simulink library "Stewart_Gough_Library"  (Simulink 7.7)
settings: Solver=ode45  StartTime=0.0  StopTime=10.0  RelTol=1e-3
undefined symbols (not defined in the file or in its folder): Aa1, Bb1, Cc1, Com1, Dd1, Dis_motor, none
libraries: simulink x13, Diamond16AT_UNAL x3, xpcseriallib x2, Stewart_Gough_Library x1
settings Model: Creator=BolivarNieto  LastModifiedBy=Edgar

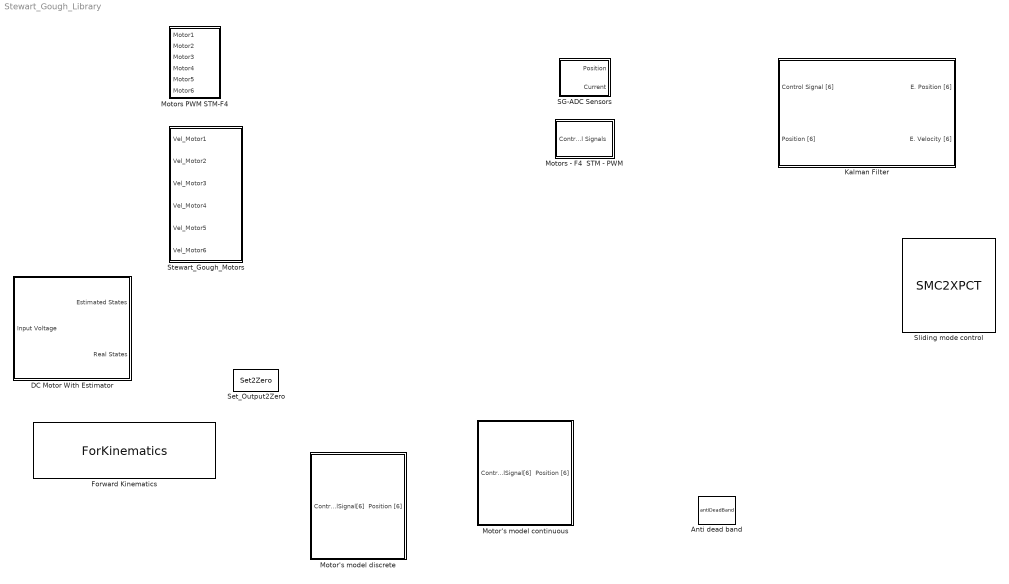
== system Stewart_Gough_Library ==
  Anti dead band : S-Function  FunctionName=antiDeadBand  Parameters=SampleTime,AntiDeadBand  EnableBusSupport=off  mask{AntiDeadBand=20, SampleTime=-1}
      mask prompts: AntiDeadBand "Anti dead band offset"; SampleTime "Sample Time (-1 inherit sample time)"
      mask Display:
      | plot([0 10],[0 10])
      | plot([10 10],[10 30])
      | plot([10 20],[30 40])
  DC Motor With Estimator : Subsystem  mask(DC Motor dynamic model){tau_m=0, kdc_m=0, iniVelo_m=0, iniPos_m=0, V_m=0}
      mask prompts: tau_m "Motor Tau"; kdc_m "Motor Kdc"; iniVelo_m "Initial Velocity"; iniPos_m "Initial Position"; V_m "Estimation Vector"
      mask help: DC Motor dynamic model with saturation, dead band, saturation, Band-Limited white noise and full state estimator
  Forward Kinematics : S-Function  FunctionName=ForKinematics  Parameters=SGini.ai,SGini.bi,ActOff  EnableBusSupport=off  mask(Forward Kinematics - Stewart Gough platform){AngBase=20, AngMobi=30, RadBase=0.150, RadMobi=0.090, ActMax=0.74676, ActMin=0.44196, ActOff=0.5486, OffZBase=0.066, OffZMobile=0.0409082}
      mask prompts: AngBase "Angle between group of joints - Base (Deg)"; AngMobi "Angle between group of joints - Mobile (Deg)"; RadBase "Radious base (m)"; RadMobi "Radious mobile (m)"; ActMax "Actuator max (m)"; ActMin "Actuator min (m)"; ActOff "Actuator Offset (m)"; OffZBase "Offset Z - Base (m)"; OffZMobile "Offset Z - Mobile (m)"
      mask init:
      | AngBase = AngBase/2;
      | 
      | tmpAnglBase = [AngBase;120-AngBase;120+AngBase;240-AngBase;240+AngBase;360-AngBase]*pi/180; %Angular arrangement of joints
      | 
      | aA = zeros(3,6);
      | for i=1:6
      |     aA(:,i)=[sin(tmpAnglBase(i))*RadBase;cos(tmpAnglBase(i))*RadBase; OffZBase];
      | end
      | 
      | AngMobi = AngMobi/2;
      | 
      | tmpAnglMobi = [60-AngMobi;60+AngMobi;180-AngMobi;180+AngMobi;300-AngMobi;300+AngMobi]*pi/180; %Angular arrangement of joints
      | 
      | bB = zeros(3,6);
      | for i=1:6
      |     bB(:,i)=[sin(tmpAnglMobi(i))*RadMobi;cos(tmpAnglMobi(i))*RadMobi; -OffZMobile];
      | end
      | 
      | SGini.ai = aA;
      | SGini.bi = bB;
      mask TabNameString: SG Parameters,SG Parameters,SG Parameters,SG Parameters,SG Parameters,SG Parameters,SG Parameters,SG Parameters,SG Parameters
      mask Display:
      | port_label('output', 1, 'Position WS [6]')
      | fprintf('OUTPUT \n UNITS: \n XYZ (mts) \n RPY (rad)')
      | port_label('input', 1, 'Position [6] (mts)')
  Kalman Filter : Subsystem  mask(Kalman filter){Qin=[2,2,2,2,2,2], Rin=[1,1,1,1,1,1]*1e-6, IniPos=[70,70,70,70,70,70], IniVel=[0,0,0,0,0,0], SamTimeKal=0.001}
      mask prompts: Qin "Covariance vector of white process noise w, Q [1x6]:"; Rin "Covariance vector of white measurement noise v, R [1x6]:"; IniPos "Vector of initial position (mm) [1x6]:"; IniVel "Vector of initial velocity (mm/s) [1x6]:"; SamTimeKal "Sample Time:"
      mask help:
      | Firgelli actuator's Kalman filter.
      |     --Q: [1x6] vector with the white process noise covariance, it is relative to R and measures the quality of the model compared to the sensor.
      |     --R: [1x6] vector with the white measurement noise covariance, it is relative to Q and measures the quality of the sensor compared to the model.
      mask init:
      | %-------------------------------Actuators' parameters
      | tau(1)=12.9;    %min
      | tau(2)=20.9;
      | tau(3)=16;
      | tau(4)=26.2;    %max
      | tau(5)=17.1;
      | tau(6)=15.2;    
      | 
      | kdc(1)=35.737;  %min
      | kdc(2)=65.089;
      | kdc(3)=51.966;
      | kdc(4)=74.788;  %max
      | kdc(5)=49.788;
      | kdc(6)=51.427;
      | 
      | %--------------------------------NUMBER OF ACTUATOR
      | i=1;
      | tauT=tau(i);
      | kdcT=kdc(i);
      | %--------------------------------Steady state representation
      | A=[0 1;0 -tauT];
      | B=[0;kdcT];
      | C=[1 0];
      | D=0;
      | G=[0;1];             %Process noise (noise at the input of the )
      | H=0;
      | 
      | Aa=A;
      | Bb=[B G];
      | Cc=C;
      | Dd=[D H];
      | 
      | Motor = ss(Aa,Bb,Cc,Dd);             %DC-Motor second order
      | %--------------------------------Kalman design
      | N=0;
      | [kest,L,P] = kalman(Motor,Qin(i),Rin(i),N);
      | KalmanDis1=c2d(kest,SamTimeKal);
      | 
      | %--------------------------------NUMBER OF ACTUATOR
      | i=2;
      | tauT=tau(i);
      | kdcT=kdc(i);
      | %--------------------------------Steady state representation
      | A=[0 1;0 -tauT];
      | B=[0;kdcT];
      | C=[1 0];
      | D=0;
      | G=[0;1];             %Process noise (noise at the input of the )
      | H=0;
      | 
      | Aa=A;
      | Bb=[B G];
      | Cc=C;
      | Dd=[D H];
      | 
      | Motor = ss(Aa,Bb,Cc,Dd);             %DC-Motor second order
      | %--------------------------------Kalman design
      | N=0;
      | [kest,L,P] = kalman(Motor,Qin(i),Rin(i),N);
      | KalmanDis2=c2d(kest,SamTimeKal);
      | 
      | %--------------------------------NUMBER OF ACTUATOR
      | i=3;
      | tauT=tau(i);
      | kdcT=kdc(i);
      | %--------------------------------Steady state representation
      | A=[0 1;0 -tauT];
      | B=[0;kdcT];
      | C=[1 0];
      | D=0;
      | G=[0;1];             %Process noise (noise at the input of the )
      | H=0;
      | 
      | Aa=A;
      | Bb=[B G];
      | Cc=C;
      | Dd=[D H];
      | 
      | Motor = ss(Aa,Bb,Cc,Dd);             %DC-Motor second order
      | %--------------------------------Kalman design
      | N=0;
      | [kest,L,P] = kalman(Motor,Qin(i),Rin(i),N);
      | KalmanDis3=c2d(kest,SamTimeKal);
      | 
      | %--------------------------------NUMBER OF ACTUATOR
      | i=4;
      | tauT=tau(i);
      | kdcT=kdc(i);
      | %--------------------------------Steady state representation
      | A=[0 1;0 -tauT];
      | B=[0;kdcT];
      | C=[1 0];
      | D=0;
      | G=[0;1];             %Process noise (noise at the input of the )
      | H=0;
      | 
      | Aa=A;
      | Bb=[B G];
      | Cc=C;
      | Dd=[D H];
      | 
      | Motor = ss(Aa,Bb,Cc,Dd);             %DC-Motor second order
      | %--------------------------------Kalman design
      | N=0;
      | [kest,L,P] = kalman(Motor,Qin(i),Rin(i),N);
      | KalmanDis4=c2d(kest,SamTimeKal);
      | 
      | %--------------------------------NUMBER OF ACTUATOR
      | i=5;
      | tauT=tau(i);
      | kdcT=kdc(i);
      | %--------------------------------Steady state representation
      | A=[0 1;0 -tauT];
      | B=[0;kdcT];
      | C=[1 0];
      | D=0;
      | G=[0;1];             %Process noise (noise at the input of the )
      | H=0;
      | 
      | Aa=A;
      | Bb=[B G];
      | Cc=C;
      | Dd=[D H];
      | 
      | Motor = ss(Aa,Bb,Cc,Dd);             %DC-Motor second order
      | %--------------------------------Kalman design
      | N=0;
      | [kest,L,P] = kalman(Motor,Qin(i),Rin(i),N);
      | KalmanDis5=c2d(kest,SamTimeKal);
      | 
      | %--------------------------------NUMBER OF ACTUATOR
      | i=6;
      | tauT=tau(i);
      | kdcT=kdc(i);
      | %--------------------------------Steady state representation
      | A=[0 1;0 -tauT];
      | B=[0;kdcT];
      | C=[1 0];
      | D=0;
      | G=[0;1];             %Process noise (noise at the input of the )
      | H=0;
      | 
      | Aa=A;
      | Bb=[B G];
      | Cc=C;
      | Dd=[D H];
      | 
      | Motor = ss(Aa,Bb,Cc,Dd);             %DC-Motor second order
      | %--------------------------------Kalman design
      | N=0;
      | [kest,L,P] = kalman(Motor,Qin(i),Rin(i),N);
      | KalmanDis6=c2d(kest,SamTimeKal);
      mask Display:
      | disp('Estimator \n Firgelli Actuator')
      | port_label('output', 1, 'E. Position [6]')
      | port_label('output', 2, 'E. Velocity [6]')
      | port_label('input', 1, 'Control Signal [6]')
      | port_label('input', 2, 'Position [6]')
  Motor's model continuous : Subsystem  mask{Taus=[12.9;20.9;16;26.2;17.1;15.2], Kdcs=[35.737; 65.089; 51.966; 74.788; 49.788; 51.427], IniPos=[70;70;70;70;70;70], IniVel=[0;0;0;0;0;0], Vmax=12}
      mask prompts: Taus "Tau:"; Kdcs "Kdc:"; IniPos "Initial Position vector:"; IniVel "Initial Velocity vector:"; Vmax "Motor peak Voltage:"
  Motor's model discrete : Subsystem  mask{Taus=[12.9;20.9;16;26.2;17.1;15.2], Kdcs=[35.737; 65.089; 51.966; 74.788; 49.788; 51.427], IniPos=[70;70;70;70;70;70], IniVel=[0;0;0;0;0;0], Vmax=12}
      mask prompts: Taus "Tau:"; Kdcs "Kdc:"; IniPos "Initial position vector:"; IniVel "Initial Velocity Vector"; Vmax "Motor peak Voltage"
      mask init:
      | for i = 1:6
      |     A = [0 1; 0 -Taus(i)];
      |     B = [0; Kdcs(i)];
      |     C = [1 0;0 1];
      |     D = [0;0];    
      |     Con_motor(:,:,i) = ss(A,B,C,D);
      |     Dis_motor(:,:,i) = c2d(Con_motor(:,:,i),0.001);
      | end
  Motors - F4  STM - PWM : Subsystem  RequirementInfo="{}  %GIDa_83dcfb88_5bb3_4bf6_bc9f_f3909d4bf5a3"
      mask Type: Protocol for PWM generation through STM-F4
      mask Description:
      | Comunication protocol for PWM generation. This block communicates a STM-F4 through serial comunication. The STM-F4 generates the PWMs required for motor control.
      | 
      | The input for this block is the percentage duty cicle for each of the six motors.
  Motors PWM STM-F4 : Subsystem  mask(Protocol for PWM generation through a STM-F4 board){Satura=80}
      mask prompts: Satura "Saturation"
      mask help:
      | Comunication protocol for PWM generation. This block communicates a STM-F4 through serial comunication. The STM-F4 generates the PWMs required for motor control.
      |
      | The input for this block is the percentage duty cicle for each of the six motors.
      mask Help: No Help!! ahhhh!!
  SG-ADC Sensors : Subsystem  mask(SG-ADC-Sensors){SamTimeADC=0.001, CutFreq=20, IniSt=[0 0 0 0 0 0]}
      mask prompts: SamTimeADC "Sample Time"; CutFreq "Cutoff frequency"; IniSt "Initial States Filter:"
      mask help: ADC from sensors, reading from I/O board daemmond 16AT and using a Discrete digital filter to remove noise.
      mask init:
      | IniStates=[0 IniSt(1)*1.4141;...
      |            0 IniSt(2)*1.4141;...
      |            0 IniSt(3)*1.4141;...
      |            0 IniSt(4)*1.4141;...
      |            0 IniSt(5)*1.4141;...
      |            0 IniSt(6)*1.4141;...                
      |            ];
      | %Filter design
      | n=2;
      | freq=1/SamTimeADC;
      | Wn=CutFreq/(freq/2);          %Sampled to 1kHz and cutof frequency of 20Hz
      | [Aa1,Bb1,Cc1,Dd1]=butter(n,Wn,'low');
      mask TabNameString: Main,Main,Main
  Set_Output2Zero : S-Function  FunctionName=Set2Zero  EnableBusSupport=off
  Sliding mode control : S-Function  FunctionName=SMC2XPCT  Parameters=eta, lambda, tau  EnableBusSupport=off  mask(Sliding mode control block){eta=0.1, lambda=1, tau=26.2}
      mask help:
      | This block implements a Sliding Mode position controler for a DC-motor.
      | It requieres the motor's position and velocity along with the desired position, velocity and aceleration.
      |
      | --Eta: Is related to a "safe factor" for stability.
      | --Lambda: Determines the rate of convergence to 0 of the error.
      | --Tau: Refers to the coeficient tau in the dinamic model.
      |
      | To change especific constants like F, please go to the "mdlOutputs" function in the c code of the S-function.
      mask Display:
      | port_label('output', 1, 'U')
      | port_label('output', 2, 'S')
      | port_label('input', 1, 'xd, xdP, xdPP')
      | port_label('input', 2, 'dm, dmP')
      | disp('SMC')
  Stewart_Gough_Motors : Subsystem  mask(Stewart Gough Motors Block  ){PWM_amp=4, PWM_freq=1000, Rpm2Pwm=1, SampleTime_ed=0.00005}
      mask prompts: PWM_amp "PWM Amplitude"; PWM_freq "PWM frequency (Hz)"; Rpm2Pwm "RPM to PWM's duty cycle gain"; SampleTime_ed "SampleTime"
      mask help: PWM Generator for 6 motors at the Stewart Gough. PWM generation is compatible with the H-Bridge 33887
      mask Help:
      | Set PWM parameters from the block dialog:
      | 
      | * PWM Amplitude stands for the amplitude when PWM is at high.
      | * RPM to PWM's duty cycle sets the conversion gain between the motor speed in RPM and the correspond duty cycle at the PWM generation.

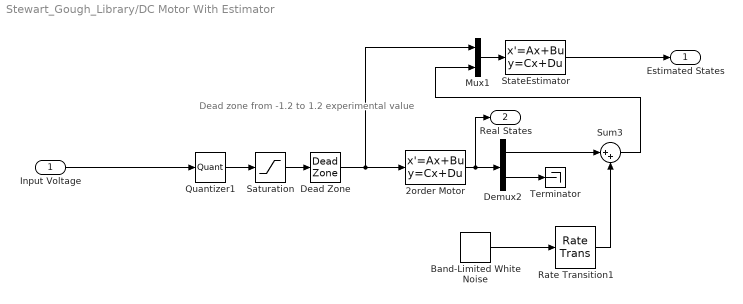
== system Stewart_Gough_Library/DC Motor With Estimator ==
  note: Dead zone from -1.2 to 1.2
      | experimental value
  Input Voltage : Inport
  2order Motor : StateSpace  A=[0 1; 0 -tau_m]  B=[0; kdc_m]  C=[1 0;0 1]  D=[0;0]  X0=[iniPos_m iniVelo_m]  ContinuousStateAttributes={'LinearPosition','LinearVelocity'}
  Band-Limited White Noise : simulink/Sources/Band-Limited White Noise  SystemSampleTime=-1  Cov=[0.0001]  Ts=0.1  seed=[23341]
  Dead Zone : DeadZone  LowerValue=0  UpperValue=0  ZeroCross=off  SaturateOnIntegerOverflow=on
  Demux2 : Demux  Outputs=2
  Mux1 : Mux  Inputs=2
  Quantizer1 : Quantizer  QuantizationInterval=0.1
  Rate Transition1 : RateTransition
  Saturation : Saturate  UpperLimit=12  LowerLimit=-12  ZeroCross=off
  StateEstimator : StateSpace  A=[-V_m(1) 1; -V_m(2) -tau_m]  B=[0 V_m(1); kdc_m V_m(2)]  C=[1 0; 0 1]  D=[0 0; 0 0]  X0=[iniPos_m iniVelo_m]  ContinuousStateAttributes={'LinearPositionEstimated','LinearVelocityEstimated'}
  Sum3 : Sum  Inputs=|++
  Terminator : Terminator
  Estimated States : Outport
  Real States : Outport  Port=2
  wires:
  Sum3/1 -> Mux1/2
  Mux1/1 -> StateEstimator/1
  Input Voltage/1 -> Quantizer1/1
  Dead Zone/1 -> 2order Motor/1, Mux1/1
  Saturation/1 -> Dead Zone/1
  Quantizer1/1 -> Saturation/1
  Rate Transition1/1 -> Sum3/2
  Band-Limited White Noise/1 -> Rate Transition1/1
  2order Motor/1 -> Demux2/1, Real States/1
  Demux2/1 -> Sum3/1
  Demux2/2 -> Terminator/1
  StateEstimator/1 -> Estimated States/1

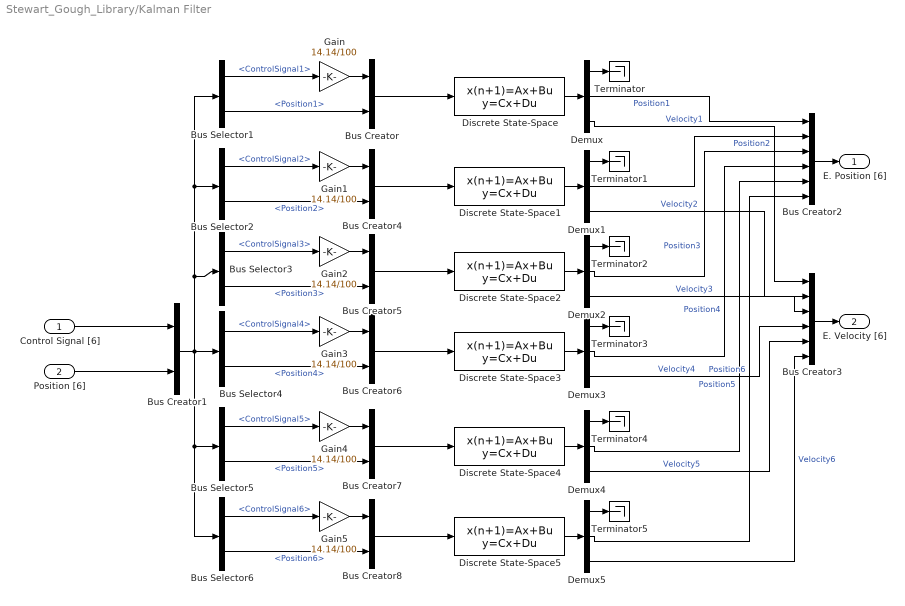
== system Stewart_Gough_Library/Kalman Filter ==
  Control Signal [6] : Inport
  Position [6] : Inport  Port=2
  Bus Creator{,1,4..8} (7 alike) : BusCreator  Inputs=2
  Bus Creator2 : BusCreator  Inputs=6
  Bus Creator3 : BusCreator  Inputs=6
  Bus Selector1 : BusSelector  OutputSignals=signal1.ControlSignal1,signal2.Position1
  Bus Selector2 : BusSelector  OutputSignals=signal1.ControlSignal2,signal2.Position2
  Bus Selector3 : BusSelector  OutputSignals=signal1.ControlSignal3,signal2.Position3
  Bus Selector4 : BusSelector  OutputSignals=signal1.ControlSignal4,signal2.Position4
  Bus Selector5 : BusSelector  OutputSignals=signal1.ControlSignal5,signal2.Position5
  Bus Selector6 : BusSelector  OutputSignals=signal1.ControlSignal6,signal2.Position6
  Demux{,1..5} (6 alike) : Demux  Outputs=3
  Discrete State-Space : DiscreteStateSpace  A=KalmanDis1.A  B=KalmanDis1.B  C=KalmanDis1.C  D=KalmanDis1.D  X0=[IniPos(1) IniVel(1)]  SampleTime=SamTimeKal
  Discrete State-Space1 : DiscreteStateSpace  A=KalmanDis2.A  B=KalmanDis2.B  C=KalmanDis2.C  D=KalmanDis2.D  X0=[IniPos(2) IniVel(2)]  SampleTime=SamTimeKal
  Discrete State-Space2 : DiscreteStateSpace  A=KalmanDis3.A  B=KalmanDis3.B  C=KalmanDis3.C  D=KalmanDis3.D  X0=[IniPos(3) IniVel(3)]  SampleTime=SamTimeKal
  Discrete State-Space3 : DiscreteStateSpace  A=KalmanDis4.A  B=KalmanDis4.B  C=KalmanDis4.C  D=KalmanDis4.D  X0=[IniPos(4) IniVel(4)]  SampleTime=SamTimeKal
  Discrete State-Space4 : DiscreteStateSpace  A=KalmanDis5.A  B=KalmanDis5.B  C=KalmanDis5.C  D=KalmanDis5.D  X0=[IniPos(5) IniVel(5)]  SampleTime=SamTimeKal
  Discrete State-Space5 : DiscreteStateSpace  A=KalmanDis6.A  B=KalmanDis6.B  C=KalmanDis6.C  D=KalmanDis6.D  X0=[IniPos(6) IniVel(6)]  SampleTime=SamTimeKal
  Gain{,1..5} (6 alike) : Gain  Gain=14.14/100
  Terminator{,1..5} (6 alike) : Terminator
  E. Position [6] : Outport
  E. Velocity [6] : Outport  Port=2
  wires:
  Bus Creator1/1 -> Bus Selector1/1, Bus Selector2/1, Bus Selector3/1, Bus Selector4/1, Bus Selector6/1, Bus Selector5/1
  Control Signal [6]/1 -> Bus Creator1/1
  Bus Creator2/1 -> E. Position [6]/1
  Position [6]/1 -> Bus Creator1/2
  Discrete State-Space/1 -> Demux/1
  Discrete State-Space1/1 -> Demux1/1
  Discrete State-Space2/1 -> Demux2/1
  Discrete State-Space3/1 -> Demux3/1
  Discrete State-Space4/1 -> Demux4/1
  Discrete State-Space5/1 -> Demux5/1
  Demux/1 -> Terminator/1
  Demux1/1 -> Terminator1/1
  Demux2/1 -> Terminator2/1
  Demux3/1 -> Terminator3/1
  Demux4/1 -> Terminator4/1
  Demux5/1 -> Terminator5/1
  Demux/2 -> Bus Creator2/1  "Position1"
  Demux1/2 -> Bus Creator2/2  "Position2"
  Demux2/2 -> Bus Creator2/3  "Position3"
  Demux3/2 -> Bus Creator2/4  "Position4"
  Demux4/2 -> Bus Creator2/5  "Position5"
  Demux5/2 -> Bus Creator2/6  "Position6"
  Bus Creator3/1 -> E. Velocity [6]/1
  Demux/3 -> Bus Creator3/1  "Velocity1"
  Demux1/3 -> Bus Creator3/2  "Velocity2"
  Demux2/3 -> Bus Creator3/3  "Velocity3"
  Demux3/3 -> Bus Creator3/4  "Velocity4"
  Demux5/3 -> Bus Creator3/6  "Velocity6"
  Demux4/3 -> Bus Creator3/5  "Velocity5"
  Bus Selector1/1 -> Gain/1  "<ControlSignal1>"
  Gain/1 -> Bus Creator/1
  Bus Selector1/2 -> Bus Creator/2  "<Position1>"
  Bus Creator/1 -> Discrete State-Space/1
  Gain1/1 -> Bus Creator4/1
  Bus Creator4/1 -> Discrete State-Space1/1
  Gain2/1 -> Bus Creator5/1
  Bus Creator5/1 -> Discrete State-Space2/1
  Gain3/1 -> Bus Creator6/1
  Gain4/1 -> Bus Creator7/1
  Gain5/1 -> Bus Creator8/1
  Bus Creator6/1 -> Discrete State-Space3/1
  Bus Creator7/1 -> Discrete State-Space4/1
  Bus Creator8/1 -> Discrete State-Space5/1
  Bus Selector2/1 -> Gain1/1  "<ControlSignal2>"
  Bus Selector2/2 -> Bus Creator4/2  "<Position2>"
  Bus Selector3/1 -> Gain2/1  "<ControlSignal3>"
  Bus Selector3/2 -> Bus Creator5/2  "<Position3>"
  Bus Selector4/1 -> Gain3/1  "<ControlSignal4>"
  Bus Selector4/2 -> Bus Creator6/2  "<Position4>"
  Bus Selector5/1 -> Gain4/1  "<ControlSignal5>"
  Bus Selector5/2 -> Bus Creator7/2  "<Position5>"
  Bus Selector6/1 -> Gain5/1  "<ControlSignal6>"
  Bus Selector6/2 -> Bus Creator8/2  "<Position6>"

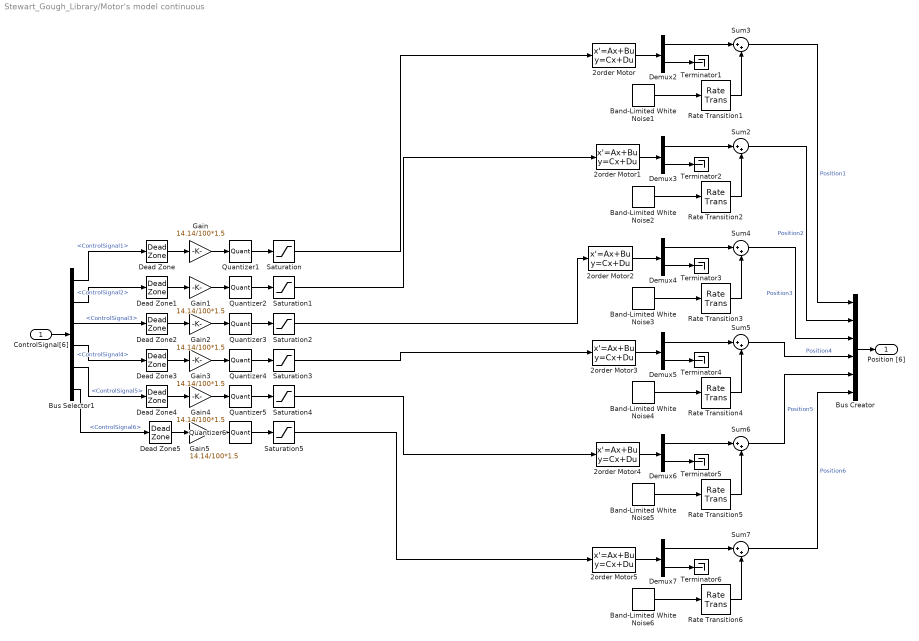
== system Stewart_Gough_Library/Motor's model continuous ==
  ControlSignal[6] : Inport
  2order Motor : StateSpace  A=[0 1; 0 -Taus(1)]  B=[0; Kdcs(1)]  C=[1 0;0 1]  D=[0;0]  X0=[IniPos(1) IniVel(1)]  ContinuousStateAttributes={'LinearPosition','LinearVelocity'}
  2order Motor1 : StateSpace  A=[0 1; 0 -Taus(2)]  B=[0; Kdcs(2)]  C=[1 0;0 1]  D=[0;0]  X0=[IniPos(2) IniVel(2)]  ContinuousStateAttributes={'LinearPosition','LinearVelocity'}
  2order Motor2 : StateSpace  A=[0 1; 0 -Taus(3)]  B=[0; Kdcs(3)]  C=[1 0;0 1]  D=[0;0]  X0=[IniPos(3) IniVel(3)]  ContinuousStateAttributes={'LinearPosition','LinearVelocity'}
  2order Motor3 : StateSpace  A=[0 1; 0 -Taus(4)]  B=[0; Kdcs(4)]  C=[1 0;0 1]  D=[0;0]  X0=[IniPos(4) IniVel(4)]  ContinuousStateAttributes={'LinearPosition','LinearVelocity'}
  2order Motor4 : StateSpace  A=[0 1; 0 -Taus(5)]  B=[0; Kdcs(5)]  C=[1 0;0 1]  D=[0;0]  X0=[IniPos(5) IniVel(5)]  ContinuousStateAttributes={'LinearPosition','LinearVelocity'}
  2order Motor5 : StateSpace  A=[0 1; 0 -Taus(6)]  B=[0; Kdcs(6)]  C=[1 0;0 1]  D=[0;0]  X0=[IniPos(6) IniVel(6)]  ContinuousStateAttributes={'LinearPosition','LinearVelocity'}
  Band-Limited White Noise{1..6} (6 alike) : simulink/Sources/Band-Limited White Noise  SystemSampleTime=-1  Cov=[0.0001]  Ts=0.1  seed=[23341]
  Bus Creator : BusCreator  Inputs=6
  Bus Selector1 : BusSelector  OutputSignals=ControlSignal1,ControlSignal2,ControlSignal3,ControlSignal4,ControlSignal5,ControlSignal6
  Dead Zone{,1..5} (6 alike) : DeadZone  LowerValue=-9.5  UpperValue=6  ZeroCross=off  SaturateOnIntegerOverflow=on
  Demux{2..7} (6 alike) : Demux  Outputs=2
  Gain{,1..5} (6 alike) : Gain  Gain=14.14/100*1.5
  Quantizer{1..6} (6 alike) : Quantizer  QuantizationInterval=0.1
  Rate Transition{1..6} (6 alike) : RateTransition
  Saturation{,1..5} (6 alike) : Saturate  UpperLimit=Vmax*1.25  LowerLimit=-Vmax*1.2  ZeroCross=off
  Sum{2..7} (6 alike) : Sum  Inputs=|++
  Terminator{1..6} (6 alike) : Terminator
  Position [6] : Outport
  wires:
  Demux2/2 -> Terminator1/1
  Demux2/1 -> Sum3/1
  2order Motor/1 -> Demux2/1
  Band-Limited White Noise1/1 -> Rate Transition1/1
  Rate Transition1/1 -> Sum3/2
  Saturation/1 -> 2order Motor/1
  Saturation2/1 -> 2order Motor2/1
  Saturation3/1 -> 2order Motor3/1
  Saturation4/1 -> 2order Motor4/1
  Saturation5/1 -> 2order Motor5/1
  Demux3/2 -> Terminator2/1
  Demux3/1 -> Sum2/1
  2order Motor1/1 -> Demux3/1
  Band-Limited White Noise2/1 -> Rate Transition2/1
  Rate Transition2/1 -> Sum2/2
  Demux4/2 -> Terminator3/1
  Demux4/1 -> Sum4/1
  2order Motor2/1 -> Demux4/1
  Band-Limited White Noise3/1 -> Rate Transition3/1
  Rate Transition3/1 -> Sum4/2
  Demux5/2 -> Terminator4/1
  Demux5/1 -> Sum5/1
  2order Motor3/1 -> Demux5/1
  Band-Limited White Noise4/1 -> Rate Transition4/1
  Rate Transition4/1 -> Sum5/2
  Demux6/2 -> Terminator5/1
  Demux6/1 -> Sum6/1
  2order Motor4/1 -> Demux6/1
  Band-Limited White Noise5/1 -> Rate Transition5/1
  Rate Transition5/1 -> Sum6/2
  Demux7/2 -> Terminator6/1
  Demux7/1 -> Sum7/1
  2order Motor5/1 -> Demux7/1
  Band-Limited White Noise6/1 -> Rate Transition6/1
  Rate Transition6/1 -> Sum7/2
  Sum3/1 -> Bus Creator/1  "Position1"
  Sum2/1 -> Bus Creator/2  "Position2"
  Sum4/1 -> Bus Creator/3  "Position3"
  Sum5/1 -> Bus Creator/4  "Position4"
  Sum6/1 -> Bus Creator/5  "Position5"
  Sum7/1 -> Bus Creator/6  "Position6"
  Bus Selector1/1 -> Dead Zone/1  "<ControlSignal1>"
  Bus Selector1/2 -> Dead Zone1/1  "<ControlSignal2>"
  Bus Selector1/3 -> Dead Zone2/1  "<ControlSignal3>"
  Bus Selector1/4 -> Dead Zone3/1  "<ControlSignal4>"
  Bus Selector1/5 -> Dead Zone4/1  "<ControlSignal5>"
  Bus Selector1/6 -> Dead Zone5/1  "<ControlSignal6>"
  ControlSignal[6]/1 -> Bus Selector1/1
  Bus Creator/1 -> Position [6]/1
  Saturation1/1 -> 2order Motor1/1
  Quantizer1/1 -> Saturation/1
  Quantizer2/1 -> Saturation1/1
  Quantizer3/1 -> Saturation2/1
  Quantizer4/1 -> Saturation3/1
  Quantizer5/1 -> Saturation4/1
  Quantizer6/1 -> Saturation5/1
  Gain/1 -> Quantizer1/1
  Gain1/1 -> Quantizer2/1
  Gain2/1 -> Quantizer3/1
  Gain3/1 -> Quantizer4/1
  Gain4/1 -> Quantizer5/1
  Gain5/1 -> Quantizer6/1
  Dead Zone1/1 -> Gain1/1
  Dead Zone2/1 -> Gain2/1
  Dead Zone3/1 -> Gain3/1
  Dead Zone4/1 -> Gain4/1
  Dead Zone5/1 -> Gain5/1
  Dead Zone/1 -> Gain/1

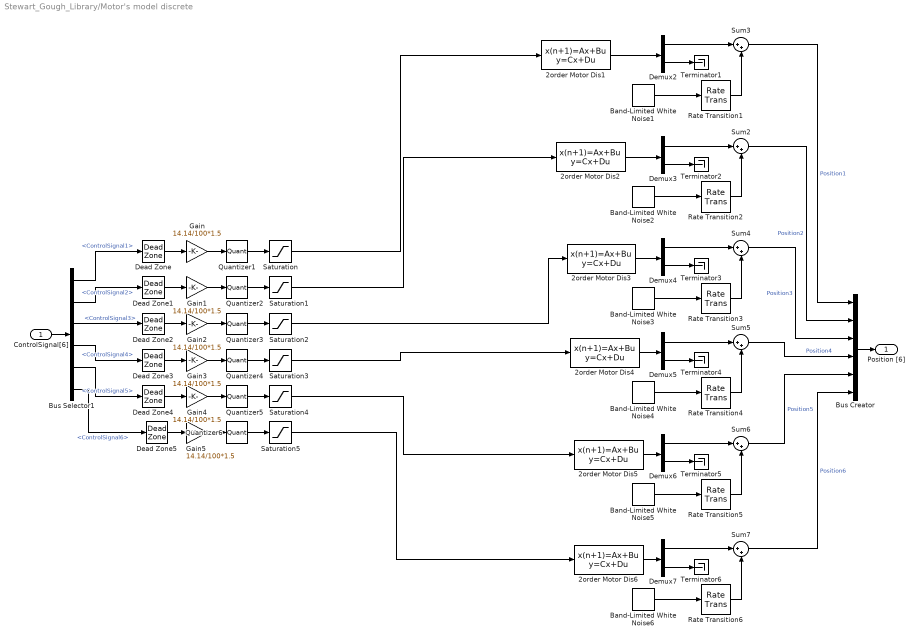
== system Stewart_Gough_Library/Motor's model discrete ==
  ControlSignal[6] : Inport
  2order Motor Dis1 : DiscreteStateSpace  A=Dis_motor(:,:,1).A  B=Dis_motor(:,:,1).B  C=Dis_motor(:,:,1).C  D=Dis_motor(:,:,1).D  X0=[IniPos(1) IniVel(1)]  SampleTime=0.001
  2order Motor Dis2 : DiscreteStateSpace  A=Dis_motor(:,:,2).A  B=Dis_motor(:,:,2).B  C=Dis_motor(:,:,2).C  D=Dis_motor(:,:,2).D  X0=[IniPos(2) IniVel(2)]  SampleTime=0.001
  2order Motor Dis3 : DiscreteStateSpace  A=Dis_motor(:,:,3).A  B=Dis_motor(:,:,3).B  C=Dis_motor(:,:,3).C  D=Dis_motor(:,:,3).D  X0=[IniPos(3) IniVel(3)]  SampleTime=0.001
  2order Motor Dis4 : DiscreteStateSpace  A=Dis_motor(:,:,4).A  B=Dis_motor(:,:,4).B  C=Dis_motor(:,:,4).C  D=Dis_motor(:,:,4).D  X0=[IniPos(4) IniVel(4)]  SampleTime=0.001
  2order Motor Dis5 : DiscreteStateSpace  A=Dis_motor(:,:,5).A  B=Dis_motor(:,:,5).B  C=Dis_motor(:,:,5).C  D=Dis_motor(:,:,5).D  X0=[IniPos(5) IniVel(5)]  SampleTime=0.001
  2order Motor Dis6 : DiscreteStateSpace  A=Dis_motor(:,:,6).A  B=Dis_motor(:,:,6).B  C=Dis_motor(:,:,6).C  D=Dis_motor(:,:,6).D  X0=[IniPos(6) IniVel(6)]  SampleTime=0.001
  Band-Limited White Noise{1..6} (6 alike) : simulink/Sources/Band-Limited White Noise  SystemSampleTime=-1  Cov=[0.0001]  Ts=0.1  seed=[23341]
  Bus Creator : BusCreator  Inputs=6
  Bus Selector1 : BusSelector  OutputSignals=ControlSignal1,ControlSignal2,ControlSignal3,ControlSignal4,ControlSignal5,ControlSignal6
  Dead Zone{,1..5} (6 alike) : DeadZone  LowerValue=-9.5  UpperValue=6  ZeroCross=off  SaturateOnIntegerOverflow=on
  Demux{2..7} (6 alike) : Demux  Outputs=2
  Gain{,1..5} (6 alike) : Gain  Gain=14.14/100*1.5
  Quantizer{1..6} (6 alike) : Quantizer  QuantizationInterval=0.1
  Rate Transition{1..6} (6 alike) : RateTransition
  Saturation{,1..5} (6 alike) : Saturate  UpperLimit=Vmax*1.25  LowerLimit=-Vmax*1.2  ZeroCross=off
  Sum{2..7} (6 alike) : Sum  Inputs=|++
  Terminator{1..6} (6 alike) : Terminator
  Position [6] : Outport
  wires:
  Demux2/2 -> Terminator1/1
  Demux2/1 -> Sum3/1
  2order Motor Dis1/1 -> Demux2/1
  Band-Limited White Noise1/1 -> Rate Transition1/1
  Rate Transition1/1 -> Sum3/2
  Quantizer1/1 -> Saturation/1
  Saturation/1 -> 2order Motor Dis1/1
  Quantizer2/1 -> Saturation1/1
  Saturation1/1 -> 2order Motor Dis2/1
  Quantizer3/1 -> Saturation2/1
  Saturation2/1 -> 2order Motor Dis3/1
  Quantizer4/1 -> Saturation3/1
  Saturation3/1 -> 2order Motor Dis4/1
  Quantizer5/1 -> Saturation4/1
  Saturation4/1 -> 2order Motor Dis5/1
  Quantizer6/1 -> Saturation5/1
  Saturation5/1 -> 2order Motor Dis6/1
  Demux3/2 -> Terminator2/1
  Demux3/1 -> Sum2/1
  2order Motor Dis2/1 -> Demux3/1
  Band-Limited White Noise2/1 -> Rate Transition2/1
  Rate Transition2/1 -> Sum2/2
  Demux4/2 -> Terminator3/1
  Demux4/1 -> Sum4/1
  2order Motor Dis3/1 -> Demux4/1
  Band-Limited White Noise3/1 -> Rate Transition3/1
  Rate Transition3/1 -> Sum4/2
  Demux5/2 -> Terminator4/1
  Demux5/1 -> Sum5/1
  2order Motor Dis4/1 -> Demux5/1
  Band-Limited White Noise4/1 -> Rate Transition4/1
  Rate Transition4/1 -> Sum5/2
  Demux6/2 -> Terminator5/1
  Demux6/1 -> Sum6/1
  2order Motor Dis5/1 -> Demux6/1
  Band-Limited White Noise5/1 -> Rate Transition5/1
  Rate Transition5/1 -> Sum6/2
  Demux7/2 -> Terminator6/1
  Demux7/1 -> Sum7/1
  Band-Limited White Noise6/1 -> Rate Transition6/1
  Rate Transition6/1 -> Sum7/2
  Sum3/1 -> Bus Creator/1  "Position1"
  Sum2/1 -> Bus Creator/2  "Position2"
  Sum4/1 -> Bus Creator/3  "Position3"
  Sum5/1 -> Bus Creator/4  "Position4"
  Sum6/1 -> Bus Creator/5  "Position5"
  Sum7/1 -> Bus Creator/6  "Position6"
  Bus Selector1/1 -> Dead Zone/1  "<ControlSignal1>"
  Bus Selector1/2 -> Dead Zone1/1  "<ControlSignal2>"
  Bus Selector1/3 -> Dead Zone2/1  "<ControlSignal3>"
  Bus Selector1/4 -> Dead Zone3/1  "<ControlSignal4>"
  Bus Selector1/5 -> Dead Zone4/1  "<ControlSignal5>"
  Bus Selector1/6 -> Dead Zone5/1  "<ControlSignal6>"
  ControlSignal[6]/1 -> Bus Selector1/1
  Bus Creator/1 -> Position [6]/1
  Gain/1 -> Quantizer1/1
  Gain1/1 -> Quantizer2/1
  Gain2/1 -> Quantizer3/1
  Gain3/1 -> Quantizer4/1
  Gain4/1 -> Quantizer5/1
  Gain5/1 -> Quantizer6/1
  2order Motor Dis6/1 -> Demux7/1
  Dead Zone1/1 -> Gain1/1
  Dead Zone2/1 -> Gain2/1
  Dead Zone3/1 -> Gain3/1
  Dead Zone4/1 -> Gain4/1
  Dead Zone5/1 -> Gain5/1
  Dead Zone/1 -> Gain/1

== system Stewart_Gough_Library/Motors - F4  STM - PWM ==
  Control Signals : Inport
  Bus Selector1 : BusSelector  OutputSignals=ControlSignal1,ControlSignal2,ControlSignal3,ControlSignal4,ControlSignal5,ControlSignal6
  Motors PWM STM-F4 : Stewart_Gough_Library/Motors PWM STM-F4  SystemSampleTime=-1  Satura=80
  wires:
  Bus Selector1/1 -> Motors PWM STM-F4/1  "<ControlSignal1>"
  Bus Selector1/2 -> Motors PWM STM-F4/2  "<ControlSignal2>"
  Bus Selector1/4 -> Motors PWM STM-F4/4  "<ControlSignal4>"
  Bus Selector1/5 -> Motors PWM STM-F4/5  "<ControlSignal5>"
  Bus Selector1/6 -> Motors PWM STM-F4/6  "<ControlSignal6>"
  Control Signals/1 -> Bus Selector1/1
  Bus Selector1/3 -> Motors PWM STM-F4/3  "<ControlSignal3>"

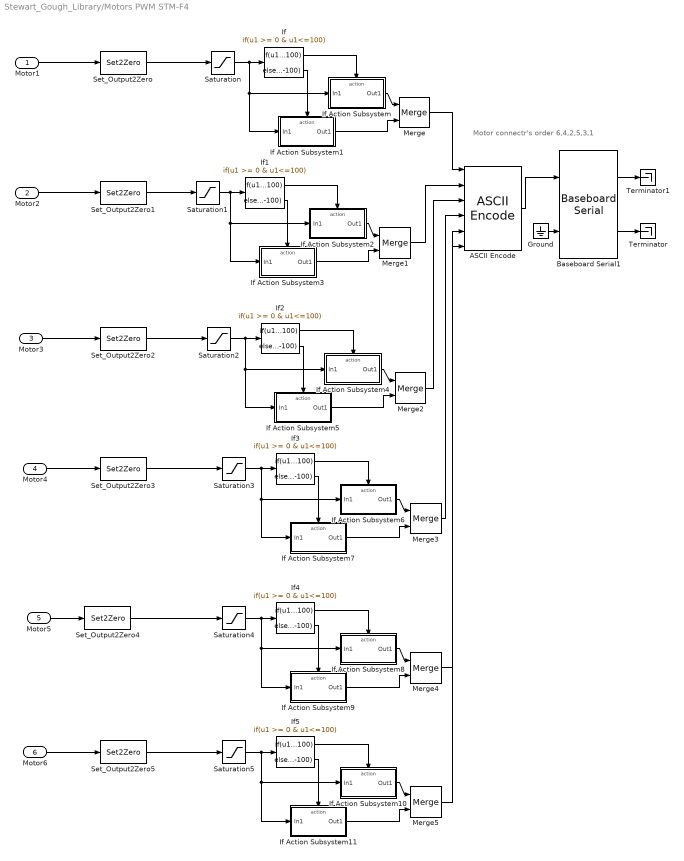
== system Stewart_Gough_Library/Motors PWM STM-F4 ==
  note: Motor connectr's order 6,4,2,5,3,1
  Motor1 : Inport
  Motor2 : Inport  Port=2
  Motor3 : Inport  Port=3
  Motor4 : Inport  Port=4
  Motor5 : Inport  Port=5
  Motor6 : Inport  Port=6
  "ASCII Encode " : xpcseriallib/ASCII Encode   format=s%c%c%c%c%c%c  nvars=6  maxlength=9  vartypes={ 'double' }
  Baseboard Serial1 : xpcseriallib/Mainboard/Baseboard Serial  SystemSampleTime=-1  group=Board Setup  port=1  irqnum=4  saddr1=0x3f8  saddr2=0x3e8  config=Com1/none  baud1=115200  parity1=None  ndata1=8  nstop1=1  fifomode1=16 deep  rlevel1=half full  automode1=off  xmtfifosize1=1024  xmtdatatype1=8 bit uint null terminated  rcvfifosize1=1024  rcvmaxread1=1024  rcvminread1=1  rcvusedelim1=on  rcvdelim1=13  rcvdatatype1=count+16 bit uint  rcvsampletime1=.001  baud2=115200  parity2=None  ndata2=8  nstop2=1  fifomode2=16 deep  rlevel2=half full  automode2=off  xmtfifosize2=1024  xmtdatatype2=8 bit uint null terminated  rcvfifosize2=1024  rcvmaxread2=1024  rcvminread2=1  rcvusedelim2=on  rcvdelim2=13  rcvdatatype2=count+16 bit uint  rcvsampletime2=.001
  Ground : Ground
  If{,1..5} (6 alike) : If  IfExpression=u1 >= 0 & u1<=100  ElseIfExpressions=u1 <0 & u1 >= -100  ShowElse=off
  If Action Subsystem : Subsystem  TreatAsAtomicUnit=on
  If Action Subsystem1 : Subsystem  TreatAsAtomicUnit=on
  If Action Subsystem10 : Subsystem  TreatAsAtomicUnit=on
  If Action Subsystem11 : Subsystem  TreatAsAtomicUnit=on
  If Action Subsystem2 : Subsystem  TreatAsAtomicUnit=on
  If Action Subsystem3 : Subsystem  TreatAsAtomicUnit=on
  If Action Subsystem4 : Subsystem  TreatAsAtomicUnit=on
  If Action Subsystem5 : Subsystem  TreatAsAtomicUnit=on
  If Action Subsystem6 : Subsystem  TreatAsAtomicUnit=on
  If Action Subsystem7 : Subsystem  TreatAsAtomicUnit=on
  If Action Subsystem8 : Subsystem  TreatAsAtomicUnit=on
  If Action Subsystem9 : Subsystem  TreatAsAtomicUnit=on
  Merge{,1..5} (6 alike) : Merge
  Saturation{,1..5} (6 alike) : Saturate  UpperLimit=Satura  LowerLimit=-Satura
  Set_Output2Zero{,1..5} (6 alike) : S-Function  FunctionName=Set2Zero  EnableBusSupport=off
  Terminator : Terminator
  Terminator1 : Terminator
  wires:
  Baseboard Serial1/2 -> Terminator/1
  If/1 -> If Action Subsystem/Action
  If/2 -> If Action Subsystem1/Action
  If Action Subsystem1/1(Out1) -> Merge/2
  If Action Subsystem/1(Out1) -> Merge/1
  Merge/1 -> "ASCII Encode "/1
  Saturation/1 -> If/1, If Action Subsystem/1(In1), If Action Subsystem1/1(In1)
  Baseboard Serial1/1 -> Terminator1/1
  If1/1 -> If Action Subsystem2/Action
  If1/2 -> If Action Subsystem3/Action
  If Action Subsystem3/1(Out1) -> Merge1/2
  If Action Subsystem2/1(Out1) -> Merge1/1
  Saturation1/1 -> If1/1, If Action Subsystem2/1(In1), If Action Subsystem3/1(In1)
  If2/1 -> If Action Subsystem4/Action
  If2/2 -> If Action Subsystem5/Action
  If Action Subsystem5/1(Out1) -> Merge2/2
  If Action Subsystem4/1(Out1) -> Merge2/1
  Saturation2/1 -> If2/1, If Action Subsystem4/1(In1), If Action Subsystem5/1(In1)
  If3/1 -> If Action Subsystem6/Action
  If3/2 -> If Action Subsystem7/Action
  If Action Subsystem7/1(Out1) -> Merge3/2
  If Action Subsystem6/1(Out1) -> Merge3/1
  Saturation3/1 -> If3/1, If Action Subsystem6/1(In1), If Action Subsystem7/1(In1)
  If4/1 -> If Action Subsystem8/Action
  If4/2 -> If Action Subsystem9/Action
  If Action Subsystem9/1(Out1) -> Merge4/2
  If Action Subsystem8/1(Out1) -> Merge4/1
  Saturation4/1 -> If4/1, If Action Subsystem8/1(In1), If Action Subsystem9/1(In1)
  If5/1 -> If Action Subsystem10/Action
  If5/2 -> If Action Subsystem11/Action
  If Action Subsystem11/1(Out1) -> Merge5/2
  If Action Subsystem10/1(Out1) -> Merge5/1
  Saturation5/1 -> If5/1, If Action Subsystem10/1(In1), If Action Subsystem11/1(In1)
  Merge1/1 -> "ASCII Encode "/2
  Merge2/1 -> "ASCII Encode "/3
  Merge3/1 -> "ASCII Encode "/4
  Merge4/1 -> "ASCII Encode "/5
  Merge5/1 -> "ASCII Encode "/6
  Motor1/1 -> Set_Output2Zero/1
  Motor2/1 -> Set_Output2Zero1/1
  Motor3/1 -> Set_Output2Zero2/1
  Motor4/1 -> Set_Output2Zero3/1
  Motor5/1 -> Set_Output2Zero4/1
  Motor6/1 -> Set_Output2Zero5/1
  Set_Output2Zero/1 -> Saturation/1
  Set_Output2Zero1/1 -> Saturation1/1
  Set_Output2Zero2/1 -> Saturation2/1
  Set_Output2Zero3/1 -> Saturation3/1
  Set_Output2Zero4/1 -> Saturation4/1
  Set_Output2Zero5/1 -> Saturation5/1
  Ground/1 -> Baseboard Serial1/2
  "ASCII Encode "/1 -> Baseboard Serial1/1

== system Stewart_Gough_Library/SG-ADC Sensors ==
  Bus Creator : BusCreator  Inputs=6
  Bus Creator3 : BusCreator  Inputs=6
  MM-16-AT Analog Input : Diamond16AT_UNAL/Diamond MM-16-AT/MM-16-AT Analog Input  RequirementInfo="{}  %GIDa_90e4469e_c027_4026_a368_80470e1f5157"  configuration=16 Single-ended  firstChan=1  numChans=12  range=0 to 10V  sampleTime=SamTimeADC  base=300
  Signal Filtering and scaling : Subsystem
  Position : Outport
  Current : Outport  Port=2
  wires:
  Signal Filtering and scaling/1(Position_1) -> Bus Creator/1  "Position1"
  Signal Filtering and scaling/2(Position_2) -> Bus Creator/2  "Position2"
  Signal Filtering and scaling/3(Position_3) -> Bus Creator/3  "Position3"
  Signal Filtering and scaling/4(Position_4) -> Bus Creator/4  "Position4"
  Signal Filtering and scaling/5(Position_5) -> Bus Creator/5  "Position5"
  Signal Filtering and scaling/6(Position_6) -> Bus Creator/6  "Position6"
  Signal Filtering and scaling/7(Current1) -> Bus Creator3/1  "Current_1"
  Signal Filtering and scaling/8(Current2) -> Bus Creator3/2  "Current_2"
  Signal Filtering and scaling/9(Current3) -> Bus Creator3/3  "Current_3"
  Signal Filtering and scaling/10(Current4) -> Bus Creator3/4  "Current_4"
  Signal Filtering and scaling/11(Current5) -> Bus Creator3/5  "Current_5"
  Signal Filtering and scaling/12(Current6) -> Bus Creator3/6  "Current_6"
  MM-16-AT Analog Input/1 -> Signal Filtering and scaling/1(In1)
  MM-16-AT Analog Input/2 -> Signal Filtering and scaling/2(In2)
  MM-16-AT Analog Input/3 -> Signal Filtering and scaling/3(In3)
  MM-16-AT Analog Input/4 -> Signal Filtering and scaling/4(In4)
  MM-16-AT Analog Input/5 -> Signal Filtering and scaling/5(In5)
  MM-16-AT Analog Input/7 -> Signal Filtering and scaling/7(In7)
  MM-16-AT Analog Input/8 -> Signal Filtering and scaling/8(In8)
  MM-16-AT Analog Input/9 -> Signal Filtering and scaling/9(In9)
  MM-16-AT Analog Input/10 -> Signal Filtering and scaling/10(In10)
  MM-16-AT Analog Input/11 -> Signal Filtering and scaling/11(In11)
  MM-16-AT Analog Input/12 -> Signal Filtering and scaling/12(In12)
  MM-16-AT Analog Input/6 -> Signal Filtering and scaling/6(In6)
  Bus Creator/1 -> Position/1
  Bus Creator3/1 -> Current/1

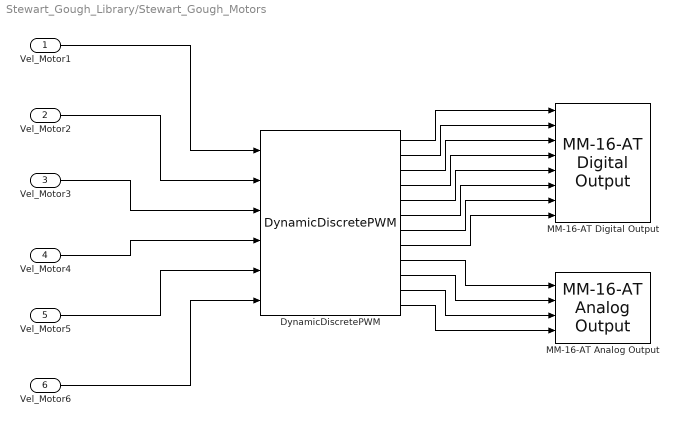
== system Stewart_Gough_Library/Stewart_Gough_Motors ==
  Vel_Motor1 : Inport
  Vel_Motor2 : Inport  Port=2
  Vel_Motor3 : Inport  Port=3
  Vel_Motor4 : Inport  Port=4
  Vel_Motor5 : Inport  Port=5
  Vel_Motor6 : Inport  Port=6
  DynamicDiscretePWM : S-Function  FunctionName=DynamicDiscretePWM  Parameters=Sample_Time,PWM_Amp,PWM_perio_Sample  EnableBusSupport=off  mask{PWM_perio=PWM_freq, PWM_Amp=PWM_amp, Sample_Time=SampleTime_ed}
      mask prompts: PWM_perio "PWM frequency (Hz)"; PWM_Amp "PWM Amplitude"; Sample_Time "Sample Time (s)"
      mask init:
      | PWM_perio_Sample=1/PWM_perio;
      | PWM_perio_Sample=round(PWM_perio_Sample/Sample_Time);
  MM-16-AT Analog Output : Diamond16AT_UNAL/Diamond MM-16-AT/MM-16-AT Analog Output  channel=[ 1 2 3 4]  range=0V to 5V  finalValuePop=Set all outputs to 0V  initValue=[0]  sampletime=SampleTime_ed  baseAddress=300
  MM-16-AT Digital Output : Diamond16AT_UNAL/Diamond MM-16-AT/MM-16-AT Digital Output  channel=[1 2 3 4 5 6 7 8]  reset=[1]  initValue=[0]  sampleTime=SampleTime_ed  baseAddress2=300
  wires:
  DynamicDiscretePWM/1 -> MM-16-AT Digital Output/1
  DynamicDiscretePWM/2 -> MM-16-AT Digital Output/2
  DynamicDiscretePWM/3 -> MM-16-AT Digital Output/3
  DynamicDiscretePWM/4 -> MM-16-AT Digital Output/4
  DynamicDiscretePWM/5 -> MM-16-AT Digital Output/5
  DynamicDiscretePWM/6 -> MM-16-AT Digital Output/6
  DynamicDiscretePWM/7 -> MM-16-AT Digital Output/7
  DynamicDiscretePWM/8 -> MM-16-AT Digital Output/8
  DynamicDiscretePWM/9 -> MM-16-AT Analog Output/1
  DynamicDiscretePWM/10 -> MM-16-AT Analog Output/2
  DynamicDiscretePWM/11 -> MM-16-AT Analog Output/3
  DynamicDiscretePWM/12 -> MM-16-AT Analog Output/4
  Vel_Motor1/1 -> DynamicDiscretePWM/1
  Vel_Motor2/1 -> DynamicDiscretePWM/2
  Vel_Motor3/1 -> DynamicDiscretePWM/3
  Vel_Motor4/1 -> DynamicDiscretePWM/4
  Vel_Motor5/1 -> DynamicDiscretePWM/5
  Vel_Motor6/1 -> DynamicDiscretePWM/6

== system Stewart_Gough_Library/Motors PWM STM-F4/If Action Subsystem ==
  In1 : Inport
  Action Port : ActionPort
  Constant8 : Constant  Value=50
  Rounding Function : Rounding  Operator=ceil
  Sum : Sum  Inputs=|++
  Out1 : Outport
  wires:
  In1/1 -> Sum/1
  Sum/1 -> Rounding Function/1
  Constant8/1 -> Sum/2
  Rounding Function/1 -> Out1/1

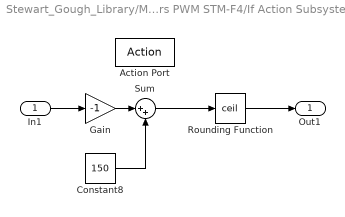
== system Stewart_Gough_Library/Motors PWM STM-F4/If Action Subsystem1 ==
  In1 : Inport
  Action Port : ActionPort
  Constant8 : Constant  Value=150
  Gain : Gain  Gain=-1
  Rounding Function : Rounding  Operator=ceil
  Sum : Sum  Inputs=|++
  Out1 : Outport
  wires:
  In1/1 -> Gain/1
  Gain/1 -> Sum/1
  Constant8/1 -> Sum/2
  Sum/1 -> Rounding Function/1
  Rounding Function/1 -> Out1/1

== system Stewart_Gough_Library/Motors PWM STM-F4/If Action Subsystem10 ==
  In1 : Inport
  Action Port : ActionPort
  Constant8 : Constant  Value=50
  Rounding Function : Rounding  Operator=ceil
  Sum : Sum  Inputs=|++
  Out1 : Outport
  wires:
  In1/1 -> Sum/1
  Sum/1 -> Rounding Function/1
  Constant8/1 -> Sum/2
  Rounding Function/1 -> Out1/1

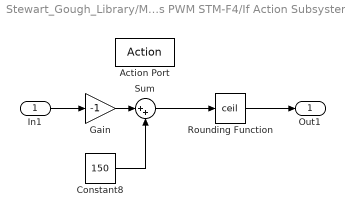
== system Stewart_Gough_Library/Motors PWM STM-F4/If Action Subsystem11 ==
  In1 : Inport
  Action Port : ActionPort
  Constant8 : Constant  Value=150
  Gain : Gain  Gain=-1
  Rounding Function : Rounding  Operator=ceil
  Sum : Sum  Inputs=|++
  Out1 : Outport
  wires:
  In1/1 -> Gain/1
  Gain/1 -> Sum/1
  Constant8/1 -> Sum/2
  Sum/1 -> Rounding Function/1
  Rounding Function/1 -> Out1/1

== system Stewart_Gough_Library/Motors PWM STM-F4/If Action Subsystem2 ==
  In1 : Inport
  Action Port : ActionPort
  Constant8 : Constant  Value=50
  Rounding Function : Rounding  Operator=ceil
  Sum : Sum  Inputs=|++
  Out1 : Outport
  wires:
  In1/1 -> Sum/1
  Sum/1 -> Rounding Function/1
  Constant8/1 -> Sum/2
  Rounding Function/1 -> Out1/1

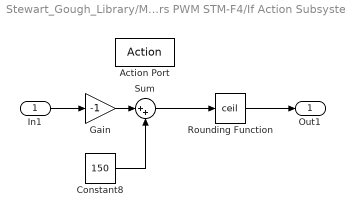
== system Stewart_Gough_Library/Motors PWM STM-F4/If Action Subsystem3 ==
  In1 : Inport
  Action Port : ActionPort
  Constant8 : Constant  Value=150
  Gain : Gain  Gain=-1
  Rounding Function : Rounding  Operator=ceil
  Sum : Sum  Inputs=|++
  Out1 : Outport
  wires:
  In1/1 -> Gain/1
  Gain/1 -> Sum/1
  Constant8/1 -> Sum/2
  Sum/1 -> Rounding Function/1
  Rounding Function/1 -> Out1/1

== system Stewart_Gough_Library/Motors PWM STM-F4/If Action Subsystem4 ==
  In1 : Inport
  Action Port : ActionPort
  Constant8 : Constant  Value=50
  Rounding Function : Rounding  Operator=ceil
  Sum : Sum  Inputs=|++
  Out1 : Outport
  wires:
  In1/1 -> Sum/1
  Sum/1 -> Rounding Function/1
  Constant8/1 -> Sum/2
  Rounding Function/1 -> Out1/1

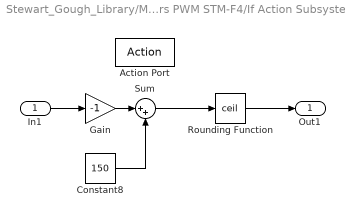
== system Stewart_Gough_Library/Motors PWM STM-F4/If Action Subsystem5 ==
  In1 : Inport
  Action Port : ActionPort
  Constant8 : Constant  Value=150
  Gain : Gain  Gain=-1
  Rounding Function : Rounding  Operator=ceil
  Sum : Sum  Inputs=|++
  Out1 : Outport
  wires:
  In1/1 -> Gain/1
  Gain/1 -> Sum/1
  Constant8/1 -> Sum/2
  Sum/1 -> Rounding Function/1
  Rounding Function/1 -> Out1/1

== system Stewart_Gough_Library/Motors PWM STM-F4/If Action Subsystem6 ==
  In1 : Inport
  Action Port : ActionPort
  Constant8 : Constant  Value=50
  Rounding Function : Rounding  Operator=ceil
  Sum : Sum  Inputs=|++
  Out1 : Outport
  wires:
  In1/1 -> Sum/1
  Sum/1 -> Rounding Function/1
  Constant8/1 -> Sum/2
  Rounding Function/1 -> Out1/1

== system Stewart_Gough_Library/Motors PWM STM-F4/If Action Subsystem7 ==
  In1 : Inport
  Action Port : ActionPort
  Constant8 : Constant  Value=150
  Gain : Gain  Gain=-1
  Rounding Function : Rounding  Operator=ceil
  Sum : Sum  Inputs=|++
  Out1 : Outport
  wires:
  In1/1 -> Gain/1
  Gain/1 -> Sum/1
  Constant8/1 -> Sum/2
  Sum/1 -> Rounding Function/1
  Rounding Function/1 -> Out1/1

== system Stewart_Gough_Library/Motors PWM STM-F4/If Action Subsystem8 ==
  In1 : Inport
  Action Port : ActionPort
  Constant8 : Constant  Value=50
  Rounding Function : Rounding  Operator=ceil
  Sum : Sum  Inputs=|++
  Out1 : Outport
  wires:
  In1/1 -> Sum/1
  Sum/1 -> Rounding Function/1
  Constant8/1 -> Sum/2
  Rounding Function/1 -> Out1/1

== system Stewart_Gough_Library/Motors PWM STM-F4/If Action Subsystem9 ==
  In1 : Inport
  Action Port : ActionPort
  Constant8 : Constant  Value=150
  Gain : Gain  Gain=-1
  Rounding Function : Rounding  Operator=ceil
  Sum : Sum  Inputs=|++
  Out1 : Outport
  wires:
  In1/1 -> Gain/1
  Gain/1 -> Sum/1
  Constant8/1 -> Sum/2
  Sum/1 -> Rounding Function/1
  Rounding Function/1 -> Out1/1

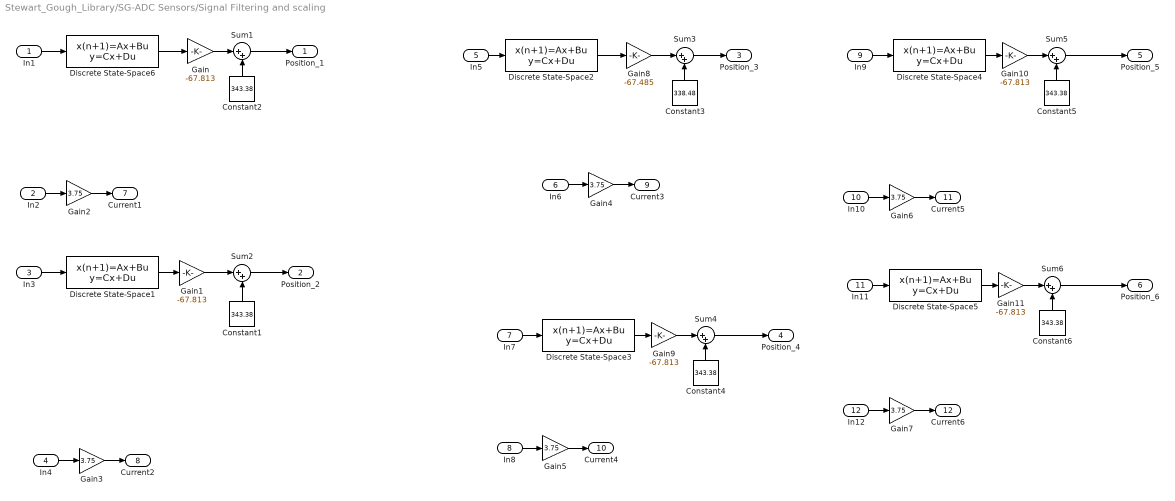
== system Stewart_Gough_Library/SG-ADC Sensors/Signal Filtering and scaling ==
  In1 : Inport
  In2 : Inport  Port=2
  In3 : Inport  Port=3
  In4 : Inport  Port=4
  In5 : Inport  Port=5
  In6 : Inport  Port=6
  In7 : Inport  Port=7
  In8 : Inport  Port=8
  In9 : Inport  Port=9
  In10 : Inport  Port=10
  In11 : Inport  Port=11
  In12 : Inport  Port=12
  Constant{1..2,4..6} (5 alike) : Constant  Value=343.38
  Constant3 : Constant  Value=338.48
  Discrete State-Space1 : DiscreteStateSpace  A=Aa1  B=Bb1  C=Cc1  D=Dd1  X0=IniStates(2,:)  SampleTime=SamTimeADC
  Discrete State-Space2 : DiscreteStateSpace  A=Aa1  B=Bb1  C=Cc1  D=Dd1  X0=IniStates(3,:)  SampleTime=SamTimeADC
  Discrete State-Space3 : DiscreteStateSpace  A=Aa1  B=Bb1  C=Cc1  D=Dd1  X0=IniStates(4,:)  SampleTime=SamTimeADC
  Discrete State-Space4 : DiscreteStateSpace  A=Aa1  B=Bb1  C=Cc1  D=Dd1  X0=IniStates(5,:)  SampleTime=SamTimeADC
  Discrete State-Space5 : DiscreteStateSpace  A=Aa1  B=Bb1  C=Cc1  D=Dd1  X0=IniStates(5,:)  SampleTime=SamTimeADC
  Discrete State-Space6 : DiscreteStateSpace  A=Aa1  B=Bb1  C=Cc1  D=Dd1  X0=IniStates(1,:)  SampleTime=SamTimeADC
  Gain{,1,9..11} (5 alike) : Gain  Gain=-67.813
  Gain{2..7} (6 alike) : Gain  Gain=3.75
  Gain8 : Gain  Gain=-67.485
  Sum{1..6} (6 alike) : Sum  Inputs=|++
  Position_1 : Outport
  Position_2 : Outport  Port=2
  Position_3 : Outport  Port=3
  Position_4 : Outport  Port=4
  Position_5 : Outport  Port=5
  Position_6 : Outport  Port=6
  Current1 : Outport  Port=7
  Current2 : Outport  Port=8
  Current3 : Outport  Port=9
  Current4 : Outport  Port=10
  Current5 : Outport  Port=11
  Current6 : Outport  Port=12
  wires:
  Constant2/1 -> Sum1/2
  Gain/1 -> Sum1/1
  In2/1 -> Gain2/1
  Gain2/1 -> Current1/1
  In4/1 -> Gain3/1
  Gain3/1 -> Current2/1
  In6/1 -> Gain4/1
  Gain4/1 -> Current3/1
  In8/1 -> Gain5/1
  Gain5/1 -> Current4/1
  In10/1 -> Gain6/1
  Gain6/1 -> Current5/1
  In12/1 -> Gain7/1
  Gain7/1 -> Current6/1
  Gain1/1 -> Sum2/1
  Constant1/1 -> Sum2/2
  Gain8/1 -> Sum3/1
  Constant3/1 -> Sum3/2
  Gain9/1 -> Sum4/1
  Constant4/1 -> Sum4/2
  Gain10/1 -> Sum5/1
  Constant5/1 -> Sum5/2
  Gain11/1 -> Sum6/1
  Constant6/1 -> Sum6/2
  In1/1 -> Discrete State-Space6/1
  Discrete State-Space6/1 -> Gain/1
  Sum1/1 -> Position_1/1
  In7/1 -> Discrete State-Space3/1
  Discrete State-Space3/1 -> Gain9/1
  Sum4/1 -> Position_4/1
  In9/1 -> Discrete State-Space4/1
  Discrete State-Space4/1 -> Gain10/1
  In11/1 -> Discrete State-Space5/1
  Discrete State-Space5/1 -> Gain11/1
  Sum6/1 -> Position_6/1
  Sum5/1 -> Position_5/1
  Sum3/1 -> Position_3/1
  Discrete State-Space2/1 -> Gain8/1
  In5/1 -> Discrete State-Space2/1
  Sum2/1 -> Position_2/1
  Discrete State-Space1/1 -> Gain1/1
  In3/1 -> Discrete State-Space1/1
